simulink model "simon"  (R2016b)
settings: Solver=ode45  StartTime=0.0  StopTime=9.58  RelTol=1e-3  EnableMultiTasking=on
values from neighbouring files (symbols this model uses):
  a = 0.1    [LoopShapingFilter.m]    (also in LoopShapingFilterNoisy.m; LoopShapingLeadCompensator.m = as(i); LoopShapingPIController.m; Untitled2.m)
  A = [0 1; 0 -c/m]    [Untitled2.m]    (also in define_consts.m; loadProperties.m; t.mat = [0  1; 0  -0.025]; test.m)
  B = [0;1/m]    [Untitled2.m]    (also in define_consts.m; loadProperties.m; t.mat = [0 0.1]; test.m = [0 0;1/m 0])
  C = [1 0]    [Untitled2.m]    (also in deadline4.m = tf([4, 1],[0, 2]); define_consts.m; loadProperties.m; t.mat)
  d = 5    [LoopShapingFilterNoisy.m]    (also in LoopShapingLeadCompensator.m = 0; define_consts.m = 0; loadProperties.m = 0)
  G0 = getGain(Hcontroller * P, wco)    [LoopShapingFilter.m]    (also in LoopShapingFilterNoisy.m; LoopShapingFinal.m = getGain(P, wco); LoopShapingLeadCompensator.m = getGain(H, wco); LoopShapingPIController.m)
  n = 0    [LoopShapingLeadCompensator.m]    (also in define_consts.m; loadProperties.m)
  wco = 5    [LoopShapingFilter.m]    (also in LoopShapingFilterNoisy.m = 3; LoopShapingFinal.m = 7.2; LoopShapingLeadCompensator.m = 7.24; LoopShapingPIController.m = 3)
  whf = 1    [LoopShapingLeadCompensator.m]    (also in loadProperties.m = 15)
  wpi = 0    [LoopShapingLeadCompensator.m]    (also in loadProperties.m = 0.1)
  x0 = [0 0]    [define_consts.m]    (also in loadProperties.m; t.mat = [1 0]; test.m; test_ref2.m = [1 0])
libraries: commchan3 x2
settings Model: Creator=Maryse Hoebeke  LastModifiedBy=Adrien
settings OptimizationCC: LifeSpan=inf
settings DebuggingCC: SFUnexpectedBacktrackingDiag=warning  SFNoUnconditionalDefaultTransitionDiag=warning  SFExecutionAtInitializationDiag=none
settings GRTTargetCC: TargetLangStandard=C89/C90 (ANSI)  GeneratePreprocessorConditionals=Disable all
settings ConfigComp: CovMetricSettings=dw  CovHtmlReporting=on  CovSaveCumulativeToWorkspaceVar=on  CovSaveSingleToWorkspaceVar=on  CovExternalEMLEnable=off

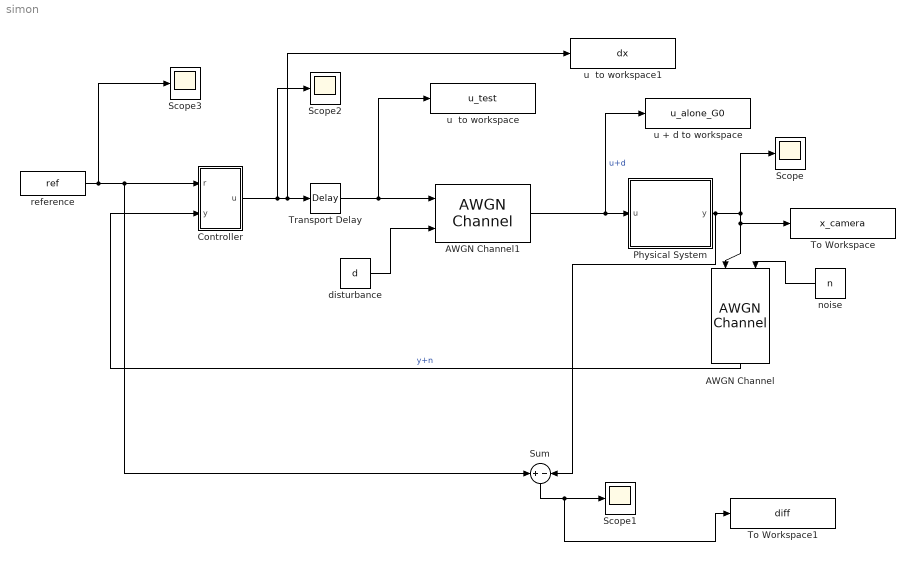
== system simon ==
  AWGN Channel : commchan3/AWGN Channel  InputProcessing=Columns as channels (frame based)  seed=67  noiseMode=Variance from port  EbNodB=10  EsNodB=10  SNRdB=10  bitsPerSym=1  Ps=1  Tsym=1  variance=1
  AWGN Channel1 : commchan3/AWGN Channel  InputProcessing=Columns as channels (frame based)  seed=67  noiseMode=Variance from port  EbNodB=10  EsNodB=10  SNRdB=10  bitsPerSym=1  Ps=1  Tsym=1  variance=1
  Controller : Subsystem
  Physical System : Subsystem
  Scope{,1..3} (4 alike) : Scope
  Sum : Sum  Inputs=+|-
  To Workspace : ToWorkspace  VariableName=x_camera  SaveFormat=Structure With Time  SampleTime=-1
  To Workspace1 : ToWorkspace  VariableName=diff  SaveFormat=Structure With Time  SampleTime=-1
  Transport Delay : TransportDelay  DelayTime=0
  disturbance : Constant  Value=d
  noise : Constant  Value=n
  reference : FromWorkspace  VariableName=ref  SampleTime=step  Interpolate=off  OutputAfterFinalValue=Holding final value
  u  to workspace : ToWorkspace  VariableName=u_test  SaveFormat=Structure With Time  SampleTime=-1
  u  to workspace1 : ToWorkspace  VariableName=dx  SaveFormat=Structure With Time  SampleTime=-1
  "u + d to workspace " : ToWorkspace  VariableName=u_alone_G0  SaveFormat=Timeseries  SampleTime=-1
  wires:
  disturbance/1 -> AWGN Channel1/2
  noise/1 -> AWGN Channel/2
  reference/1 -> Scope3/1, Sum/1, Controller/1(r)
  AWGN Channel/1 -> Controller/2(y)  "y+n"
  Controller/1(u) -> Scope2/1, u  to workspace1/1, Transport Delay/1
  Physical System/1(y) -> Sum/2, Scope/1, To Workspace/1, AWGN Channel/1
  Sum/1 -> To Workspace1/1, Scope1/1
  AWGN Channel1/1 -> "u + d to workspace "/1, Physical System/1(u)  "u+d"
  Transport Delay/1 -> u  to workspace/1, AWGN Channel1/1

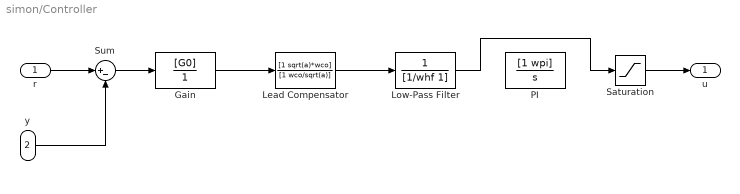
== system simon/Controller ==
  r : Inport
  y : Inport  Port=2
  Gain : TransferFcn  Numerator=[G0]  Denominator=[1]
  Lead Compensator : TransferFcn  Numerator=[1 sqrt(a)*wco]  Denominator=[1 wco/sqrt(a)]
  Low-Pass Filter : TransferFcn  Denominator=[1/whf 1]
  PI : TransferFcn  Numerator=[1 wpi]  Denominator=[1 0]
  Saturation : Saturate  UpperLimit=70  LowerLimit=-70
  Sum : Sum  Inputs=|+-
  u : Outport
  wires:
  r/1 -> Sum/1
  y/1 -> Sum/2
  Saturation/1 -> u/1
  Sum/1 -> Gain/1
  Gain/1 -> Lead Compensator/1
  Lead Compensator/1 -> Low-Pass Filter/1
  Low-Pass Filter/1 -> Saturation/1

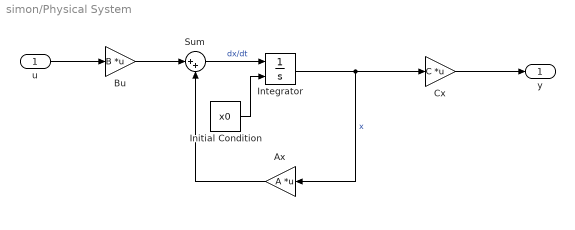
== system simon/Physical System ==
  u : Inport
  Ax : Gain  Gain=A  Multiplication=Matrix(K*u)
  Bu : Gain  Gain=B  Multiplication=Matrix(K*u)
  Cx : Gain  Gain=C  Multiplication=Matrix(K*u)
  Initial Condition : Constant  Value=x0
  Integrator : Integrator  InitialConditionSource=external  InitialCondition=x0
  Sum : Sum  Inputs=|++
  y : Outport
  wires:
  Integrator/1 -> Cx/1, Ax/1  "x"
  Initial Condition/1 -> Integrator/2
  Cx/1 -> y/1
  Bu/1 -> Sum/1
  u/1 -> Bu/1
  Ax/1 -> Sum/2
  Sum/1 -> Integrator/1  "dx/dt"
